simulink model "TwoLoopAdaptiveNeuralNetworkBasedController"  (R2020b)
settings: Solver=ode4  StartTime=0.0  StopTime=100.0  FixedStep=1e-3  RelTol=1e-3
settings Model: Creator=Ivan Lopez  LastModifiedBy=Ivan Lopez

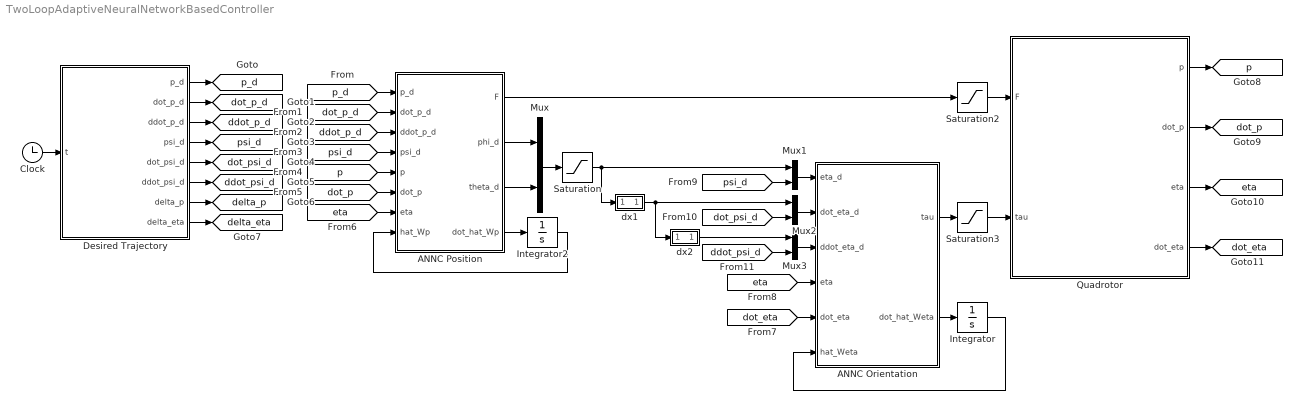
== system TwoLoopAdaptiveNeuralNetworkBasedController ==
  ANNC Orientation : MATLAB Function  TreatAsAtomicUnit=on
  ANNC Position : MATLAB Function  TreatAsAtomicUnit=on
  Clock : Clock
  Desired Trajectory : MATLAB Function  TreatAsAtomicUnit=on
  Integrator : Integrator  InitialCondition=zeros(10,3)
  Integrator2 : Integrator  InitialCondition=zeros(10,3)
  Mux{,1..3} (4 alike) : Mux  Inputs=2
  Quadrotor : Subsystem
  Saturation : Saturate  UpperLimit=20*pi/180  LowerLimit=-20*pi/180
  Saturation2 : Saturate  UpperLimit=34.4  LowerLimit=0
  Saturation3 : Saturate  UpperLimit=1.72  LowerLimit=-1.72
  dx1 : Subsystem
  dx2 : Subsystem
  tag scope: ddot_p_d=global, ddot_psi_d=global, delta_eta=global, delta_p=global, dot_eta=global, dot_p=global, dot_p_d=global, dot_psi_d=global, eta=global, p=global, p_d=global, psi_d=global
  wires:
  Desired Trajectory/8(delta_eta) -> [delta_eta]
  Desired Trajectory/1(p_d) -> [p_d]
  Desired Trajectory/3(ddot_p_d) -> [ddot_p_d]
  Desired Trajectory/5(dot_psi_d) -> [dot_psi_d]
  Desired Trajectory/7(delta_p) -> [delta_p]
  Desired Trajectory/6(ddot_psi_d) -> [ddot_psi_d]
  Desired Trajectory/4(psi_d) -> [psi_d]
  Clock/1 -> Desired Trajectory/1(t)
  Desired Trajectory/2(dot_p_d) -> [dot_p_d]
  [ddot_psi_d] -> Mux3/2
  Mux1/1 -> ANNC Orientation/1(eta_d)
  Mux2/1 -> ANNC Orientation/2(dot_eta_d)
  [psi_d] -> Mux1/2
  ANNC Position/3(theta_d) -> Mux/2
  Saturation/1 -> Mux1/1, dx1/1(x)
  Mux3/1 -> ANNC Orientation/3(ddot_eta_d)
  Mux/1 -> Saturation/1
  [dot_psi_d] -> Mux2/2
  dx1/1(dx) -> dx2/1(x), Mux2/1
  ANNC Position/2(phi_d) -> Mux/1
  dx2/1(dx) -> Mux3/1
  Quadrotor/2(dot_p) -> [dot_p]
  Quadrotor/4(dot_eta) -> [dot_eta]
  Quadrotor/3(eta) -> [eta]
  Quadrotor/1(p) -> [p]
  ANNC Position/4(dot_hat_Wp) -> Integrator2/1
  Integrator2/1 -> ANNC Position/8(hat_Wp)
  [p_d] -> ANNC Position/1(p_d)
  [dot_p_d] -> ANNC Position/2(dot_p_d)
  [ddot_p_d] -> ANNC Position/3(ddot_p_d)
  [psi_d] -> ANNC Position/4(psi_d)
  [p] -> ANNC Position/5(p)
  [dot_p] -> ANNC Position/6(dot_p)
  [eta] -> ANNC Position/7(eta)
  [eta] -> ANNC Orientation/4(eta)
  [dot_eta] -> ANNC Orientation/5(dot_eta)
  ANNC Orientation/2(dot_hat_Weta) -> Integrator/1
  Integrator/1 -> ANNC Orientation/6(hat_Weta)
  ANNC Orientation/1(tau) -> Saturation3/1
  ANNC Position/1(F) -> Saturation2/1
  Saturation2/1 -> Quadrotor/1(F)
  Saturation3/1 -> Quadrotor/2(tau)

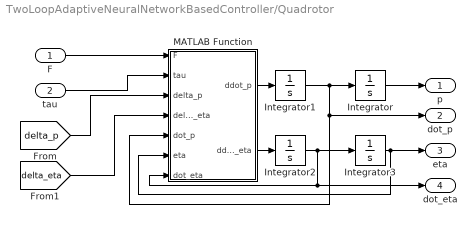
== system TwoLoopAdaptiveNeuralNetworkBasedController/Quadrotor ==
  F : Inport
  tau : Inport  Port=2
  Integrator : Integrator  InitialCondition=[0;0;0.3]  LimitOutput=on  UpperSaturationLimit=[inf;inf;inf]  LowerSaturationLimit=[-inf;-inf;0.3]
  Integrator1 : Integrator  InitialCondition=[0;0;0]
  Integrator2 : Integrator  InitialCondition=[0;0;0]
  Integrator3 : Integrator  InitialCondition=[0;0;0]  LimitOutput=on  UpperSaturationLimit=[pi/2; pi/2; inf]  LowerSaturationLimit=[-pi/2; -pi/2; -inf]
  MATLAB Function : MATLAB Function  TreatAsAtomicUnit=on
  p : Outport
  dot_p : Outport  Port=2
  eta : Outport  Port=3
  dot_eta : Outport  Port=4
  wires:
  [delta_p] -> MATLAB Function/3(delta_p)
  [delta_eta] -> MATLAB Function/4(delta_eta)
  F/1 -> MATLAB Function/1(F)
  Integrator3/1 -> MATLAB Function/6(eta), eta/1
  Integrator1/1 -> dot_p/1, MATLAB Function/5(dot_p), Integrator/1
  MATLAB Function/2(ddot_eta) -> Integrator2/1
  MATLAB Function/1(ddot_p) -> Integrator1/1
  tau/1 -> MATLAB Function/2(tau)
  Integrator2/1 -> Integrator3/1, dot_eta/1, MATLAB Function/7(dot_eta)
  Integrator/1 -> p/1

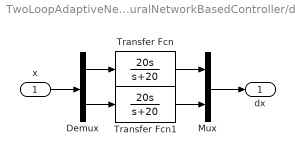
== system TwoLoopAdaptiveNeuralNetworkBasedController/dx1 ==
  x : Inport
  Demux : Demux  Outputs=2
  Mux : Mux  Inputs=2
  Transfer Fcn : TransferFcn  Numerator=[20 0]  Denominator=[1 20]
  Transfer Fcn1 : TransferFcn  Numerator=[20 0]  Denominator=[1 20]
  dx : Outport
  wires:
  Demux/2 -> Transfer Fcn1/1
  Demux/1 -> Transfer Fcn/1
  Transfer Fcn/1 -> Mux/1
  Transfer Fcn1/1 -> Mux/2
  Mux/1 -> dx/1
  x/1 -> Demux/1

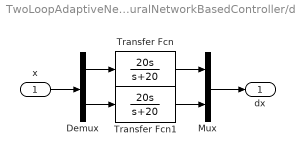
== system TwoLoopAdaptiveNeuralNetworkBasedController/dx2 ==
  x : Inport
  Demux : Demux  Outputs=2
  Mux : Mux  Inputs=2
  Transfer Fcn : TransferFcn  Numerator=[20 0]  Denominator=[1 20]
  Transfer Fcn1 : TransferFcn  Numerator=[20 0]  Denominator=[1 20]
  dx : Outport
  wires:
  x/1 -> Demux/1
  Mux/1 -> dx/1
  Transfer Fcn1/1 -> Mux/2
  Transfer Fcn/1 -> Mux/1
  Demux/1 -> Transfer Fcn/1
  Demux/2 -> Transfer Fcn1/1

== matlab function TwoLoopAdaptiveNeuralNetworkBasedController/Quadrotor/MATLAB Function ==
  data: F input; ddot_p output; ddot_eta output; tau input; delta_p input; delta_eta input; dot_p input; eta input; dot_eta input
function [ddot_p, ddot_eta] = fcn(F, tau, delta_p, delta_eta, dot_p, eta, dot_eta)

m  = 1.79;
g  = 9.81;
Ixx = 0.03; Iyy = 0.03; Izz = 0.04;
dx = 0.002; dy = 0.002; dz = 0.004;
d_phi = 0.002; d_theta = 0.002; d_psi = 0.004;
I  = diag([Ixx Iyy Izz]);
Dp = diag([dx dy dz]);
Dn = diag([d_phi d_theta d_psi]);
Vz = [0; 0; 1];

phi     = eta(1);     theta     = eta(2);     psi = eta(3);
dot_phi = dot_eta(1); dot_theta = dot_eta(2);

R = [cos(theta)*cos(psi)  sin(phi)*sin(theta)*cos(psi)-cos(phi)*sin(psi)  cos(phi)*sin(theta)*cos(psi)+sin(phi)*sin(psi)
     cos(theta)*sin(psi)  sin(phi)*sin(theta)*sin(psi)+cos(phi)*cos(psi)  cos(phi)*sin(theta)*sin(psi)-sin(phi)*cos(psi)
     -sin(theta)          sin(phi)*cos(theta)                             cos(phi)*cos(theta)];
 
% W = [1  sin(phi)*tan(theta)  cos(phi)*tan(theta)
%      0  cos(phi)             -sin(phi)
%      0  sin(phi)/cos(theta)  cos(phi)/cos(theta)];

iW = [1 0         -sin(theta)
      0 cos(phi)  cos(theta)*sin(phi)
      0 -sin(phi) cos(theta)*cos(phi)];
 
dot_W = [0  (cos(phi)*tan(theta))+((sin(phi)*dot_theta)/(cos(theta)^2))                     ((cos(phi)*dot_theta)/(cos(theta)^2))-(sin(phi)*tan(theta)*dot_phi)
         0  -sin(phi)*dot_phi                                                               -cos(phi)*dot_phi
         0  ((cos(phi)*cos(theta)*dot_phi)+(sin(phi)*sin(theta)*dot_theta))/(cos(theta)^2)  ((cos(phi)*sin(theta)*dot_theta)-(sin(phi)*cos(theta)*dot_phi))/(cos(theta)^2)];
  
iWdot_eta = iW*dot_eta;

SiWdot_eta = [0              -iWdot_eta(3)  iWdot_eta(2)
              iWdot_eta(3)   0              -iWdot_eta(1)
              -iWdot_eta(2)  iWdot_eta(1)   0];

M = iW'*I*iW;
C = iW'*(SiWdot_eta*I - I*iW*dot_W)*iW;

ddot_p   = (R*Vz*F + delta_p - m*g*Vz - Dp*dot_p)/m;
ddot_eta = M\(iW'*tau + delta_eta - C*dot_eta - Dn*dot_eta);

== matlab function TwoLoopAdaptiveNeuralNetworkBasedController/Desired Trajectory ==
  data: t input; p_d output; dot_p_d output; ddot_p_d output; psi_d output; dot_psi_d output; ddot_psi_d output; delta_p output; delta_eta output
function [p_d, dot_p_d, ddot_p_d, psi_d, dot_psi_d, ddot_psi_d, delta_p, delta_eta] = fcn(t)
z0    = 0.3;
h     = 1.4;
%% Circunferencia
% ampx = 1;
% ampy = 1;
% ampz = 0.1;
% amps = 10*pi/180;
% frecx = 2*pi/5;
% frecy = 2*pi/5;
% frecz = 2*pi/5;
% frecs = 2*pi/5;

%% Lemniscata 1
% 
% ampx = 0.5;
% ampy = 1;
% ampz = 0.4;
% amps = 5*pi/180;
% frecx = 2*pi/4;
% frecy = 2*pi/8;
% frecz = 2*pi/4;
% frecs = 2*pi/4;
% 
% x_d      = ampx*sin(frecx*t);
% dot_x_d  = ampx*frecx*cos(frecx*t);
% ddot_x_d = -ampx*frecx^2*sin(frecx*t);
% 
% y_d      = ampy*cos(frecy*t);
% dot_y_d  = -ampy*frecy*sin(frecy*t);
% ddot_y_d = -ampy*frecy^2*cos(frecy*t);
% 
% if (t>=0 && t<=5)
%     z_d      = h - (h - z0)*exp(-ampz*t^3);
%     dot_z_d  = 3*ampz*t^2*(h - z0)*exp(-ampz*t^3);
%     ddot_z_d = (3*ampz*t^3 - 2)*3*ampz*t*(z0 - h)*exp(-ampz*t^3);
% else
%     z_d      = (h - ampz) + ampz*sin(frecz*t);
%     dot_z_d  = ampz*frecz*cos(frecz*t);
%     ddot_z_d = -ampz*frecz^2*sin(frecz*t);
% end
% 
% psi_d      = [amps*sin(frecs*t)
%               amps*frecs*cos(frecs*t)
%              -amps*frecs^2*sin(frecs*t)];
%        
% p_d      = [x_d; y_d; z_d];
% dot_p_d  = [dot_x_d; dot_y_d; dot_z_d];
% ddot_p_d = [ddot_x_d; ddot_y_d; ddot_z_d];

%% Lemniscata 2 (Experimento)

ampx = 0.5;
ampy = 1;
frecx = 2*pi/4;
frecy = 2*pi/8;
frecz = 2*pi/4;

x_d      = ampx*sin(frecx*t);
dot_x_d  = ampx*frecx*cos(frecx*t);
ddot_x_d = -ampx*frecx^2*sin(frecx*t);

y_d      = ampy*cos(frecy*t);
dot_y_d  = -ampy*frecy*sin(frecy*t);
ddot_y_d = -ampy*frecy^2*cos(frecy*t);

if (t>=0 && t<=5)
    z_d      = 1 - 0.7*exp(-0.1*t^3);
    dot_z_d  = 0.3*t^2*0.7*exp(-0.1*t^3);
    ddot_z_d = 0.3*0.7*(-0.1*3*exp(-0.1*t^3)*t^4 + 2*exp(-0.1*t^3)*t);
else
    z_d      = 1;
    dot_z_d  = 0;
    ddot_z_d = 0;
end

psi_d      = 0;
dot_psi_d  = 0;
ddot_psi_d = 0;
       
p_d      = [x_d; y_d; z_d];
dot_p_d  = [dot_x_d; dot_y_d; dot_z_d];
ddot_p_d = [ddot_x_d; ddot_y_d; ddot_z_d];

%% Disturbances
if (t>=60)
    delta_p = [0.5*sin(2*frecx*t)
               0.5*cos(2*frecy*t)
               0.5*sin(2*frecz*t)];

    d_eta = 0.045*sin(2.5*pi*t-3) + 0.09*sin(2*pi*t-7) + 0.135*sin(0.5*pi*t-9.5) + 0.09*sin(0.3*pi*t) + 0.054*sin(0.15*pi*t+4.5) + 0.045*sin(0.05*pi*t+2) + 0.135*sin(0.01*pi*t+3) + 0.225;
    delta_eta = [d_eta; d_eta; d_eta];
else
    delta_p = [0;0;0];
    delta_eta = [0;0;0];
end

== matlab function TwoLoopAdaptiveNeuralNetworkBasedController/ANNC Position ==
  data: p_d input; F output; dot_p_d input; ddot_p_d input; psi_d input; p input; dot_p input; eta input; phi_d output; theta_d output; dot_hat_Wp output; hat_Wp input
function [F, phi_d, theta_d, dot_hat_Wp] = fcn(p_d, dot_p_d, ddot_p_d, psi_d, p, dot_p, eta, hat_Wp)
m       = 1.79;
g       = 9.81;
gz      = [0; 0; g];
phi     = eta(1);
theta   = eta(2);
e_p     = p_d - p;
dot_e_p = dot_p_d - dot_p;
%% Position controller %%%
%%% Gains %%%
hat_m = 0.85*m; % mass uncertainty
KUp   = diag([0.75 0.75 10]);
Kp    = diag([1.75 1.75 12]);

Up       = dot_p_d + Kp*e_p;
dot_Up   = ddot_p_d + Kp*dot_e_p;
tilde_Up = Up - dot_p;
%%% Neural Network Structure %%%
gamma_p   = [1; dot_p; eta; dot_Up];
neurons_p = 10;
V_p = [0.6294   -0.0292    0.4863   -0.9311    0.3102    0.9186    0.2321   -0.8921   -0.6687    0.9923
    0.8116    0.6006   -0.2155   -0.1225   -0.6748    0.0944   -0.0534    0.0616    0.2040   -0.8436
   -0.7460   -0.7162    0.3110   -0.2369   -0.7620   -0.7228   -0.2967    0.5583   -0.4741   -0.1146
    0.8268   -0.1565   -0.6576    0.5310   -0.0033   -0.7014    0.6617    0.8680    0.3082   -0.7867
    0.2647    0.8315    0.4121    0.5904    0.9195   -0.4850    0.1705   -0.7402    0.3784    0.9238
   -0.8049    0.5844   -0.9363   -0.6263   -0.3192    0.6814    0.0994    0.1376    0.4963   -0.9907
   -0.4430    0.9190   -0.4462   -0.0205    0.1705   -0.4914    0.8344   -0.0612   -0.0989    0.5498
    0.0938    0.3115   -0.9077   -0.1088   -0.5524    0.6286   -0.4283   -0.9762   -0.8324    0.6346
    0.9150   -0.9286   -0.8057    0.2926    0.5025   -0.5130    0.5144   -0.3258   -0.5420    0.7374
    0.9298    0.6983    0.6469    0.4187   -0.4898    0.8585    0.5075   -0.6756    0.8267   -0.8311];
sigma_p = tanh(V_p'*gamma_p);
%%% Neural Network Gains %%%
flag_NN = 1; % <------------ On/Off NN
N_p     = 0.85*eye(neurons_p);   % 2   % 3.5 % 2.2  % 2.2 % 2.2  % 0.65
kp      = 0.001;                 % 0.1 % 0.4 % 1.25 % 1.2 % 1.15 % 0.001
a_p     = 0.001*diag([1 1 1]);
%%% Controller %%%
F_p        = hat_m*(dot_Up + gz) + KUp*tilde_Up + flag_NN*(hat_Wp'*sigma_p + a_p*sign(tilde_Up));
dot_hat_Wp = N_p*(sigma_p*tilde_Up' - kp*norm(tilde_Up)*hat_Wp);
theta_d    = atan((F_p(1)*cos(psi_d) + F_p(2)*sin(psi_d))/F_p(3));
phi_d      = atan(cos(theta_d)*(F_p(1)*sin(psi_d) - F_p(2)*cos(psi_d))/F_p(3));
F          = F_p(3)/(cos(phi)*cos(theta));

== matlab function TwoLoopAdaptiveNeuralNetworkBasedController/ANNC Orientation ==
  settings: updateMethod=DISCRETE
  data: eta_d input; tau output; dot_eta_d input; ddot_eta_d input; eta input; dot_eta input; hat_Weta input; dot_hat_Weta output
function [tau, dot_hat_Weta] = fcn(eta_d, dot_eta_d, ddot_eta_d, eta, dot_eta, hat_Weta)

phi = eta(1) ; theta = eta(2);
%% Gains
K_Ueta = 2*diag([1 1 1]);
K_eta  = 5*diag([1 1 1]);
%% Attitude Controller
e_eta     = eta_d - eta;
dot_e_eta = dot_eta_d - dot_eta;

Ueta       = dot_eta_d + K_eta*e_eta;
dot_Ueta   = ddot_eta_d + K_eta*dot_e_eta;
tilde_Ueta = Ueta - dot_eta;

gamma_eta = [1; eta; dot_eta; dot_Ueta; K_Ueta*tilde_Ueta];
neurons_eta = 10;
V_eta = [0.6294   -0.0292    0.4863   -0.9311    0.3102    0.9186    0.2321   -0.8921   -0.6687    0.9923
    0.8116    0.6006   -0.2155   -0.1225   -0.6748    0.0944   -0.0534    0.0616    0.2040   -0.8436
   -0.7460   -0.7162    0.3110   -0.2369   -0.7620   -0.7228   -0.2967    0.5583   -0.4741   -0.1146
    0.8268   -0.1565   -0.6576    0.5310   -0.0033   -0.7014    0.6617    0.8680    0.3082   -0.7867
    0.2647    0.8315    0.4121    0.5904    0.9195   -0.4850    0.1705   -0.7402    0.3784    0.9238
   -0.8049    0.5844   -0.9363   -0.6263   -0.3192    0.6814    0.0994    0.1376    0.4963   -0.9907
   -0.4430    0.9190   -0.4462   -0.0205    0.1705   -0.4914    0.8344   -0.0612   -0.0989    0.5498
    0.0938    0.3115   -0.9077   -0.1088   -0.5524    0.6286   -0.4283   -0.9762   -0.8324    0.6346
    0.9150   -0.9286   -0.8057    0.2926    0.5025   -0.5130    0.5144   -0.3258   -0.5420    0.7374
    0.9298    0.6983    0.6469    0.4187   -0.4898    0.8585    0.5075   -0.6756    0.8267   -0.8311
   -0.6848    0.8680    0.3897    0.5094    0.0119   -0.3000   -0.2391    0.5886   -0.6952   -0.2004
    0.9412    0.3575   -0.3658   -0.4479    0.3982   -0.6068    0.1356   -0.3776    0.6516   -0.4803
    0.9143    0.5155    0.9004    0.3594    0.7818   -0.4978   -0.8483    0.0571    0.0767    0.6001];

sigma_eta = tanh(V_eta'*gamma_eta);
N_eta = 1.85*eye(neurons_eta);% 22  % 22   % 12   % 30
keta  = 0.003;                % 3.9 % 3.95 % 3.95 % 3.95
a_eta = 0.001*diag([1 1 1]);

W = [1  sin(phi)*tan(theta)  cos(phi)*tan(theta)
     0  cos(phi)             -sin(phi)
     0  sin(phi)/cos(theta)  cos(phi)/cos(theta)];

tau_eta = hat_Weta'*sigma_eta + a_eta*sign(tilde_Ueta);
tau     = W'*tau_eta;
dot_hat_Weta = N_eta*(sigma_eta*tilde_Ueta' - keta*norm(tilde_Ueta)*hat_Weta);
